simulink subsystem "ControlSample"  (R2019b)
settings: Solver=VariableStepAuto  StartTime=0.0  StopTime=10.0  RelTol=1e-3
undefined symbols (not defined in the file or in its folder): __PRM__SERIALIZED__DATA__, SubsystemReferenceBlock
settings Model: Creator=VM  LastModifiedBy=VM

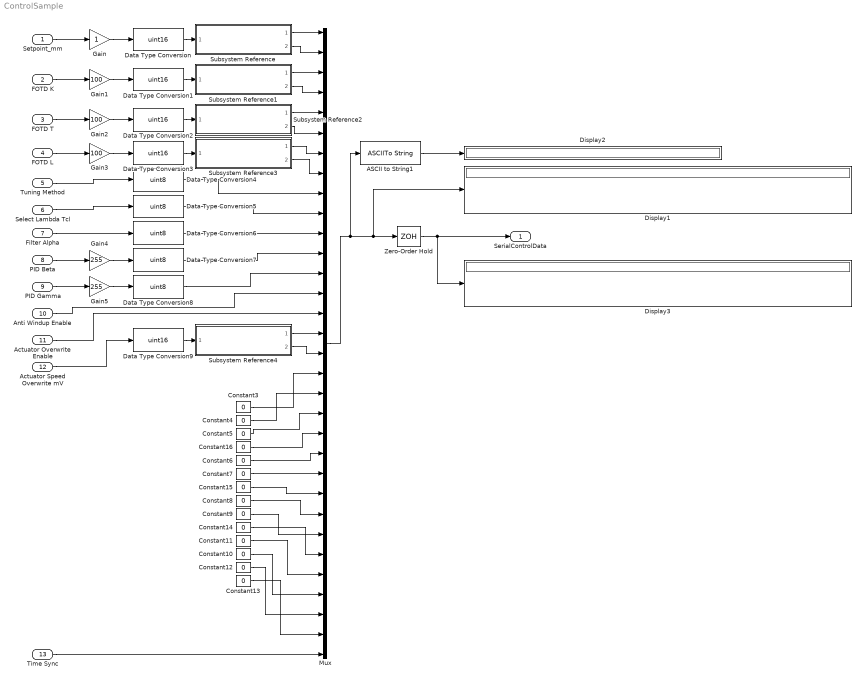
== system ControlSample ==
  Setpoint_mm : Inport
  FOTD K : Inport  Port=2
  FOTD T : Inport  Port=3
  FOTD L : Inport  Port=4
  Tuning Method : Inport  Port=5
  Select Lambda Tcl : Inport  Port=6
  Filter Alpha : Inport  Port=7
  PID Beta : Inport  Port=8
  PID Gamma : Inport  Port=9
  Anti Windup Enable : Inport  Port=10
  Actuator Overwrite Enable : Inport  Port=11
  Actuator Speed Overwrite mV : Inport  Port=12
  Time Sync : Inport  Port=13
  ASCII to String1 : ASCIIToString
  Constant{3..16} (14 alike) : Constant  Value=0  OutDataTypeStr=uint8
  Data Type Conversion{,1..3,9} (5 alike) : DataTypeConversion  OutDataTypeStr=uint16
  Data Type Conversion{4..8} (5 alike) : DataTypeConversion  OutDataTypeStr=uint8
  Display1 : Display
      settings: Decimation=32
  Display2 : Display
  Display3 : Display
      settings: Decimation=32
  Gain : Gain
  Gain1 : Gain  Gain=100
  Gain2 : Gain  Gain=100
  Gain3 : Gain  Gain=100
  Gain4 : Gain  Gain=255
  Gain5 : Gain  Gain=255
  Mux : Mux  Inputs=32
  Subsystem Reference{,1..4} (5 alike) : Subsystem  BlockKeywords=__PRM__SERIALIZED__DATA__:SubsystemReferenceBlock  ReferencedSubsystem=SerializeUINT16
  Zero-Order Hold : ZeroOrderHold  SampleTime=0.005
  SerialControlData : Outport
  wires:
  Subsystem Reference/1 -> Mux/1
  Subsystem Reference/2 -> Mux/2
  Data Type Conversion/1 -> Subsystem Reference/1
  Gain/1 -> Data Type Conversion/1
  Setpoint_mm/1 -> Gain/1
  Gain1/1 -> Data Type Conversion1/1
  Data Type Conversion1/1 -> Subsystem Reference1/1
  Subsystem Reference1/1 -> Mux/3
  Subsystem Reference1/2 -> Mux/4
  Gain2/1 -> Data Type Conversion2/1
  Data Type Conversion2/1 -> Subsystem Reference2/1
  Subsystem Reference2/1 -> Mux/5
  Subsystem Reference2/2 -> Mux/6
  Gain3/1 -> Data Type Conversion3/1
  Data Type Conversion3/1 -> Subsystem Reference3/1
  Subsystem Reference3/1 -> Mux/7
  Subsystem Reference3/2 -> Mux/8
  FOTD K/1 -> Gain1/1
  FOTD T/1 -> Gain2/1
  FOTD L/1 -> Gain3/1
  Tuning Method/1 -> Data Type Conversion4/1
  Data Type Conversion4/1 -> Mux/9
  Select Lambda Tcl/1 -> Data Type Conversion5/1
  Filter Alpha/1 -> Data Type Conversion6/1
  Data Type Conversion5/1 -> Mux/10
  Data Type Conversion6/1 -> Mux/11
  Data Type Conversion7/1 -> Mux/12
  Data Type Conversion8/1 -> Mux/13
  ASCII to String1/1 -> Display2/1
  Mux/1 -> Display1/1, Zero-Order Hold/1, ASCII to String1/1
  PID Beta/1 -> Gain4/1
  Gain4/1 -> Data Type Conversion7/1
  PID Gamma/1 -> Gain5/1
  Gain5/1 -> Data Type Conversion8/1
  Time Sync/1 -> Mux/32
  Constant3/1 -> Mux/18
  Constant4/1 -> Mux/19
  Constant5/1 -> Mux/20
  Constant6/1 -> Mux/22
  Constant7/1 -> Mux/23
  Constant8/1 -> Mux/25
  Constant9/1 -> Mux/26
  Constant10/1 -> Mux/29
  Constant11/1 -> Mux/28
  Constant12/1 -> Mux/30
  Constant13/1 -> Mux/31
  Constant15/1 -> Mux/24
  Constant16/1 -> Mux/21
  Constant14/1 -> Mux/27
  Data Type Conversion9/1 -> Subsystem Reference4/1
  Actuator Speed Overwrite mV/1 -> Data Type Conversion9/1
  Zero-Order Hold/1 -> SerialControlData/1, Display3/1
  Subsystem Reference4/1 -> Mux/16
  Subsystem Reference4/2 -> Mux/17
  Actuator Overwrite Enable/1 -> Mux/15
  Anti Windup Enable/1 -> Mux/14
